simulink library "threeOneThreeSurfaceCtrl_cl"  (R2018b)
settings: Solver=VariableStepAuto  StartTime=0.0  StopTime=10.0  RelTol=1e-3
undefined symbols (not defined in the file or in its folder): ctrl
libraries: filteredPIDController_ul x2
settings Model: Creator=mcobb  LastModifiedBy=mcobb

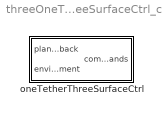
== system threeOneThreeSurfaceCtrl_cl ==
  oneTetherThreeSurfaceCtrl : Subsystem  VariantControl=VSS_controller_oneTetherThreeSurfaceCtrl

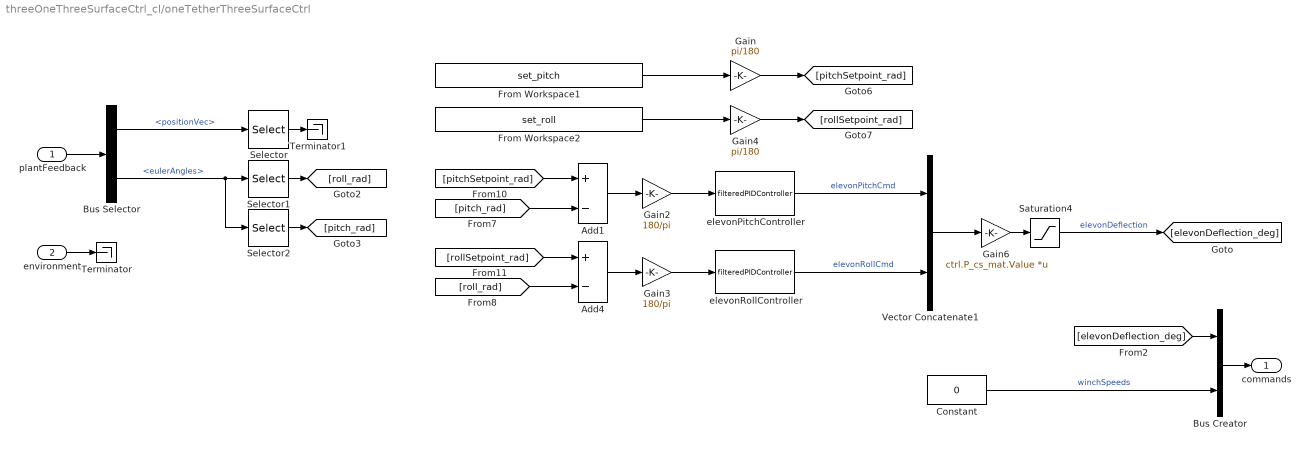
== system threeOneThreeSurfaceCtrl_cl/oneTetherThreeSurfaceCtrl ==
  plantFeedback : Inport  OutDataTypeStr=Bus: plantBus
  environment : Inport  Port=2  OutDataTypeStr=Bus: envBus
  Add1 : Sum  Inputs=+-
  Add4 : Sum  Inputs=+-
  Bus Creator : BusCreator  Inputs=2
  Bus Selector : BusSelector  OutputSignals=positionVec,eulerAngles
  Constant : Constant  Value=0
  From Workspace1 : FromWorkspace  VariableName=set_pitch  SampleTime=0
  From Workspace2 : FromWorkspace  VariableName=set_roll  SampleTime=0
  Gain : Gain  Gain=pi/180
  Gain2 : Gain  Gain=180/pi
  Gain3 : Gain  Gain=180/pi
  Gain4 : Gain  Gain=pi/180
  Gain6 : Gain  Gain=ctrl.P_cs_mat.Value  Multiplication=Matrix(K*u)
  Saturation4 : Saturate  UpperLimit=ctrl.elevon_max_deflection.Value  LowerLimit=-ctrl.elevon_max_deflection.Value
  Selector : Selector  InputPortWidth=3  IndexOptions=Index vector (dialog)  Indices=3  OutputSizes=1
  Selector1 : Selector  InputPortWidth=3  IndexOptions=Index vector (dialog)  Indices=1  OutputSizes=1
  Selector2 : Selector  InputPortWidth=3  IndexOptions=Index vector (dialog)  Indices=2  OutputSizes=1
  Terminator : Terminator
  Terminator1 : Terminator
  Vector Concatenate1 : Concatenate
  elevonPitchController : filteredPIDController_ul/filteredPIDController  kp=ctrl.elevonPitchKp.Value  ki=ctrl.elevonPitchKi.Value  kd=ctrl.elevonPitchKd.Value  Value=ctrl.elevonPitchTau.Value
  elevonRollController : filteredPIDController_ul/filteredPIDController  kp=ctrl.elevonRollKp.Value  ki=ctrl.elevonRollKi.Value  kd=ctrl.elevonRollKd.Value  Value=ctrl.elevonRollTau.Value
  commands : Outport  OutDataTypeStr=Bus: ctrlBus
  wires:
  Saturation4/1 -> [elevonDeflection_deg]  "elevonDeflection"
  Vector Concatenate1/1 -> Gain6/1
  elevonRollController/1 -> Vector Concatenate1/2  "elevonRollCmd"
  elevonPitchController/1 -> Vector Concatenate1/1  "elevonPitchCmd"
  [roll_rad] -> Add4/2
  Add4/1 -> Gain3/1
  [pitch_rad] -> Add1/2
  Gain6/1 -> Saturation4/1
  Gain2/1 -> elevonPitchController/1
  Gain3/1 -> elevonRollController/1
  Add1/1 -> Gain2/1
  Bus Creator/1 -> commands/1
  [elevonDeflection_deg] -> Bus Creator/1
  Constant/1 -> Bus Creator/2  "winchSpeeds"
  environment/1 -> Terminator/1
  plantFeedback/1 -> Bus Selector/1
  Gain/1 -> [pitchSetpoint_rad]
  Gain4/1 -> [rollSetpoint_rad]
  Selector/1 -> Terminator1/1
  [pitchSetpoint_rad] -> Add1/1
  [rollSetpoint_rad] -> Add4/1
  Bus Selector/1 -> Selector/1  "<positionVec>"
  Bus Selector/2 -> Selector2/1, Selector1/1  "<eulerAngles>"
  Selector1/1 -> [roll_rad]
  Selector2/1 -> [pitch_rad]
  From Workspace1/1 -> Gain/1
  From Workspace2/1 -> Gain4/1
